simulink library "sm_interface_elements_lib"  (R2021b)
settings: Solver=VariableStepAuto  StartTime=0.0  StopTime=10.0  RelTol=1e-3
libraries: fl_lib x6, sm_lib x6
settings Model: Creator=The MathWorks, Inc.  LastModifiedBy=The MathWorks, Inc.
settings SolverCC: AlgebraicLoopSolver=TrustRegion
settings DebuggingCC: SFMachineParentedDataDiag=warning

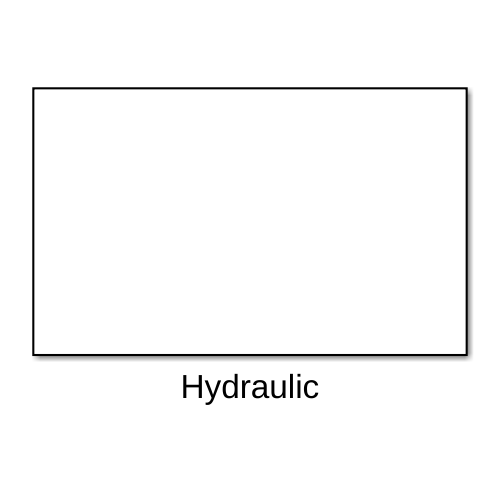
[thumbnail: Simulink's stored preview of the top-level diagram]
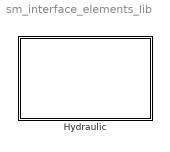
== system sm_interface_elements_lib ==
  Hydraulic : Subsystem
      mask init:
      | %

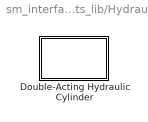
== system sm_interface_elements_lib/Hydraulic ==
  Double-Acting Hydraulic Cylinder : Subsystem  mask{barrelLength=0.5, barrelInnerRadius=0.08, barrelOuterRadius=0.1, barrelDensity=8050, barrelColor=[0.5 0.5 0.5], barrelOpacity=0.3, pistonThickness=0.05, pistonDensity=8050, pistonColor=[0.9 0.9 0.9], rodLength=0.5, rodRadius=0.04, rodDensity=8050, rodColor=[0.9 0.9 0.9], bottomCapThickness=0.05, bottomCapDensity=8050, bottomCapColor=[0.5 0.5 0.5], headCapThickness=0.05, headCapDensity=8050, headCapColor=[0.5 0.5 0.5], deadVolume_bottom=1e-6, deadVolume_head=1e-6, k_bottom=1e9, b_bottom=1500, k_head=1e9, b_head=1500, b=1e6, PositionTargetSpecify=on, PositionTargetPriority=Low (approximate), totalLength0=0.75, p0_bottom=4e6, p0_head=4e6}
      mask prompts: barrelLength "Length (m)"; barrelInnerRadius "Inner radius (m)"; barrelOuterRadius "Outer radius (m)"; barrelDensity "Density (kg/m^3)"; barrelColor "Color [R G B]"; barrelOpacity "Opacity"; pistonThickness "Thickness (m)"; pistonDensity "Density (kg/m^3)"; pistonColor "Color [R G B]"; rodLength "Length (m)"; rodRadius "Radius (m)"; rodDensity "Density (kg/m^3)"; rodColor "Color [R G B]"; bottomCapThickness "Thickness (m)"; bottomCapDensity "Density (kg/m^3)"; bottomCapColor "Color [R G B]"; headCapThickness "Thickness (m)"; headCapDensity "Density (kg/m^3)"; headCapColor "Color [R G B]"; deadVolume_bottom "Dead volume (m^3)"; deadVolume_head "Dead volume (m^3)"; k_bottom "Stiffness (N/m)"; b_bottom "Damping (N/(m/s))"; k_head "Stiffness (N/m)"; b_head "Damping (N/(m/s))"; b "Damping coefficient (N/m/s))"; PositionTargetSpecify "Specify end-to-end distance"; PositionTargetPriority "Priority"; totalLength0 "Bottom outer face to rod outer face distance (m)"; p0_bottom "Bottom chamber (Pa)"; p0_head "Head chamber (Pa)"
      mask help: This block represents a double-acting single-rod hydraulic cylinder. The 'head' end of the cylinder corresponds to the side through which the piston rod emerges. The block contains Simscape Multibody frame ports at the two ends: one attached to the outer face of the bottom end cap (FB) and the other attached to the outer face of the piston rod (FR). Hydraulic conserving ports are attached to the bottom chamber (HB) and the head chamber (HH).
      mask init:
      | blk = gcb;
      | 
      | % Piston face areas
      | pistonArea_bottom = pi*barrelInnerRadius^2;
      | pistonArea_head = pi*(barrelInnerRadius^2-rodRadius^2);
      | 
      | % Cylinder barrel cross section
      | barrelCrossSection = [...
      |     barrelInnerRadius,  barrelLength/2;...
      |     barrelInnerRadius, -barrelLength/2;...
      |     barrelOuterRadius, -barrelLength/2;...
      |     barrelOuterRadius,  barrelLength/2];
      | 
      | % Cylinder head cap cross section
      | headCapCrossSection = [...
      |     rodRadius,          headCapThickness/2;...
      |     rodRadius,         -headCapThickness/2;...
      |     barrelOuterRadius, -headCapThickness/2;...
      |     barrelOuterRadius,  headCapThickness/2];
      | 
      | % Set position target on Prismatic Joint
      | if PositionTargetSpecify
      |     set_param([blk,'/Mechanical System/Prismatic Joint'],'PositionTargetSpecify', 'on');
      |     length0_bottom = totalLength0 - rodLength - pistonThickness - bottomCapThickness;
      |     set_param([blk,'/Mechanical System/Prismatic Joint'],'PositionTargetValue', num2str(length0_bottom));
      |     switch PositionTargetPriority
      |         case 1 %'Low (approximate)'
      |             set_param([blk,'/Mechanical System/Prismatic Joint'],'PositionTargetPriority','Low');
      |         case 2 %'High (desired)'
      |             set_param([blk,'/Mechanical System/Prismatic Joint'],'PositionTargetPriority','High');
      |         otherwise
      |             disp('invalid target piority setting')
      |     end
      | else
      |     length0_bottom = 0;
      |     set_param([blk,'/Mechanical System/Prismatic Joint'],'PositionTargetSpecify', 'off');
      | end
      mask Callback PositionTargetSpecify:
      | simmechanics_demohelpers_dump_trailer_temp_mo = get_param(gcb,'MaskObject');
      | simmechanics_demohelpers_dump_trailer_temp_dc = simmechanics_demohelpers_dump_trailer_temp_mo.getDialogControl('PositionTargetParams');
      | if strcmp(get_param(gcb,'PositionTargetSpecify'),'on')
      |     simmechanics_demohelpers_dump_trailer_temp_dc.Visible = 'on';
      | else
      |     simmechanics_demohelpers_dump_trailer_temp_dc.Visible = 'off';
      | end
      | clear simmechanics_demohelpers_dump_trailer_temp_mo
      | clear simmechanics_demohelpers_dump_trailer_temp_dc
      mask TypeOptions PositionTargetPriority: Low (approximate) | High (desired)
      mask DialogControl Container4 Prompt: Bodies
      mask DialogControl Container30 Prompt: Cylinder Barrel
      mask DialogControl Container34 Prompt: Piston
      mask DialogControl Container35 Prompt: Rod
      mask DialogControl Container32 Prompt: Bottom Cap
      mask DialogControl Container33 Prompt: Head Cap
      mask DialogControl Container14 Prompt: Chambers
      mask DialogControl Container28 Prompt: Bottom
      mask DialogControl Container31 Prompt: Head
      mask DialogControl Container19 Prompt: Internal Mechanics
      mask DialogControl Container38 Prompt: Bottom Stop
      mask DialogControl Container41 Prompt: Head Stop
      mask DialogControl Container37 Prompt: Viscous Friction
      mask DialogControl Container25 Prompt: Initial Conditions
      mask DialogControl Container39 Prompt: Configuration
      mask DialogControl Container40 Prompt: Pressure
      mask Display: image(fullfile(matlabroot,'toolbox','physmod','sm','smdemos','interface_elements','images','sm_interface_elements_hydraulic_cylinder.svg'));

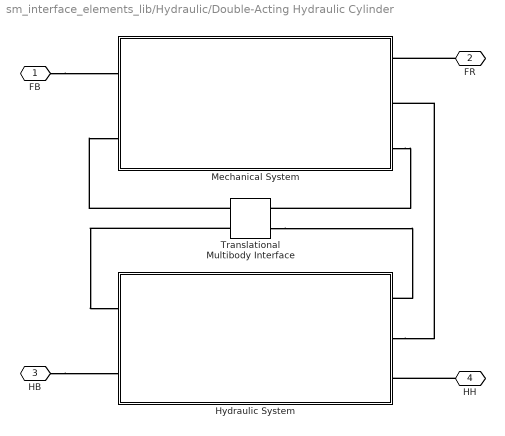
== system sm_interface_elements_lib/Hydraulic/Double-Acting Hydraulic Cylinder ==
  Hydraulic System : Subsystem
      mask Display: image(fullfile(matlabroot,'toolbox','physmod','sm','smdemos','dump_trailer','images','sm_dump_trailer_hydraulic_cylinder_hydraulic_system.svg'));
  Mechanical System : Subsystem
      mask Display: image(fullfile(matlabroot,'toolbox','physmod','sm','smdemos','dump_trailer','images','sm_dump_trailer_hydraulic_cylinder_mechanical_system.svg'));
  Translational Multibody Interface : fl_lib/Mechanical/Multibody Interfaces/Translational Multibody Interface
      settings: SourceProductBaseCode=SS
  FB : PMIOPort  Side=Left
  FR : PMIOPort  Port=2  Side=Right
  HB : PMIOPort  Port=3  Side=Left
  HH : PMIOPort  Port=4  Side=Right
  connections:
  FB/RConn1 -- Mechanical System/LConn1
  FR/RConn1 -- Mechanical System/RConn1
  HB/RConn1 -- Hydraulic System/LConn2
  HH/RConn1 -- Hydraulic System/RConn3
  Hydraulic System/RConn2 -- Mechanical System/RConn2
  Mechanical System/RConn3 -- Translational Multibody Interface/RConn1
  Translational Multibody Interface/LConn1 -- Mechanical System/LConn2
  Translational Multibody Interface/LConn2 -- Hydraulic System/LConn1
  Translational Multibody Interface/RConn2 -- Hydraulic System/RConn1

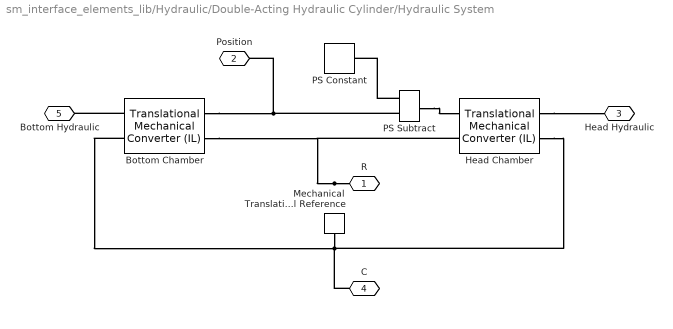
== system sm_interface_elements_lib/Hydraulic/Double-Acting Hydraulic Cylinder/Hydraulic System ==
  Bottom Chamber : fl_lib/Isothermal Liquid/Elements/Translational Mechanical Converter (IL)  mech_orientation=foundation.enum.MechOrientationTranslational.Positive  displacement_spec=foundation.enum.DisplacementSpec.InputSignal  x0=0 m  interface_area=pistonArea_bottom m^2  dead_volume=deadVolume_bottom m^3  pressure_spec=foundation.enum.pressure_spec.atmospheric  environment_pressure=0.101325 MPa  dynamic_compressibility=simscape.enum.onoff.on  p0=p0_bottom Pa
      settings: SourceProductBaseCode=SS  InternalSimscapePortConfiguration="{\"Bottom\":[],\"Left\":[{\"id\":\"A\",\"label\":\"A\",\"type\":\"foundation.isothermal_liquid.isothermal_liquid\"},{\"id\":\"C\",\"label\":\"C\",\"type\":\"foundation.mechanical.translational.translational\"}],\"Right\":[{\"id\":\"p_in\",\"label\":\"p\",\"type\":\"input\"},{\"id\":\"R\",\"label\":\"R\",\"type\":\"foundation.mechanical.translational.translational\"}],\"Top\":[]}"
  Head Chamber : fl_lib/Isothermal Liquid/Elements/Translational Mechanical Converter (IL)  mech_orientation=foundation.enum.MechOrientationTranslational.Negative  displacement_spec=foundation.enum.DisplacementSpec.InputSignal  x0=0 m  interface_area=pistonArea_head m^2  dead_volume=deadVolume_head m^3  pressure_spec=foundation.enum.pressure_spec.atmospheric  environment_pressure=0.101325 MPa  dynamic_compressibility=simscape.enum.onoff.on  p0=p0_head Pa
      settings: SourceProductBaseCode=SS  InternalSimscapePortConfiguration="{\"Bottom\":[],\"Left\":[{\"id\":\"A\",\"label\":\"A\",\"type\":\"foundation.isothermal_liquid.isothermal_liquid\"},{\"id\":\"C\",\"label\":\"C\",\"type\":\"foundation.mechanical.translational.translational\"}],\"Right\":[{\"id\":\"p_in\",\"label\":\"p\",\"type\":\"input\"},{\"id\":\"R\",\"label\":\"R\",\"type\":\"foundation.mechanical.translational.translational\"}],\"Top\":[]}"
  Mechanical Translational Reference : fl_lib/Mechanical/Translational Elements/Mechanical Translational Reference
  PS Constant : fl_lib/Physical Signals/Sources/PS Constant  constant=barrelLength-pistonThickness m
  PS Subtract : fl_lib/Physical Signals/Functions/PS Subtract
  R : PMIOPort  Side=Right
  Position : PMIOPort  Port=2  Side=Right
  Head Hydraulic : PMIOPort  Port=3  Side=Right
  C : PMIOPort  Port=4  Side=Left
  Bottom Hydraulic : PMIOPort  Port=5  Side=Left
  connections:
  Bottom Chamber/LConn1 -- Bottom Hydraulic/RConn1
  Head Chamber/LConn1 -- Head Hydraulic/RConn1
  PS Subtract/RConn1 -- Head Chamber/RConn1
  PS Subtract/LConn2 -- PS Constant/RConn1
  R/RConn1 -- Head Chamber/RConn2 -- Bottom Chamber/RConn2
  C/RConn1 -- Head Chamber/LConn2 -- Bottom Chamber/LConn2 -- Mechanical Translational Reference/LConn1
  Bottom Chamber/RConn1 -- PS Subtract/LConn1 -- Position/RConn1

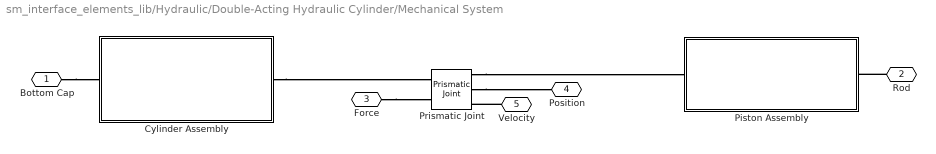
== system sm_interface_elements_lib/Hydraulic/Double-Acting Hydraulic Cylinder/Mechanical System ==
  Cylinder Assembly : Subsystem
      mask Display: image(fullfile(matlabroot,'toolbox','physmod','sm','smdemos','interface_elements','images','sm_interface_elements_hydraulic_cylinder_cylinder.png'));
  Piston Assembly : Subsystem
      mask Display: image(fullfile(matlabroot,'toolbox','physmod','sm','smdemos','interface_elements','images','sm_interface_elements_hydraulic_cylinder_piston.png'));
  Prismatic Joint : sm_lib/Joints/Prismatic Joint  JointMode=Normal  SenseConstraintForce=off  SenseConstraintForceX=off  SenseConstraintForceY=off  SenseConstraintForceZ=off  SenseConstraintTorque=off  SenseConstraintTorqueX=off  SenseConstraintTorqueY=off  SenseConstraintTorqueZ=off  SenseTotalForce=off  SenseTotalForceX=off  SenseTotalForceY=off  SenseTotalForceZ=off  SenseTotalTorque=off  SenseTotalTorqueX=off  SenseTotalTorqueY=off  SenseTotalTorqueZ=off  CompositeWrenchDir=FollowerOnBase  CompositeWrenchFrame=BaseFrame  EquilibriumPosition=0  EquilibriumPositionUnits=m  SpringStiffness=10  SpringStiffnessUnits=N/m  DampingCoefficient=b  DampingCoefficientUnits=N/(m/s)  TorqueActuationMode=InputTorque  MotionActuationMode=ComputedMotion  SensePosition=on  SenseVelocity=on  SenseAcceleration=off  SenseTorqueForce=off  SenseLowerLimitTorqueForce=off  SenseUpperLimitTorqueForce=off  LowerLimitSpecify=on  LowerLimitBound=0  LowerLimitBoundUnits=m  LowerLimitStiffness=k_bottom  LowerLimitStiffnessUnits=N/m  LowerLimitDamping=b_bottom  LowerLimitDampingUnits=N/(m/s)  LowerLimitTransitionRegionWidth=1e-4  LowerLimitTransitionRegionWidthUnits=m  UpperLimitSpecify=on  UpperLimitBound=barrelLength-pistonThickness  UpperLimitBoundUnits=m  UpperLimitStiffness=k_head  UpperLimitStiffnessUnits=N/m  UpperLimitDamping=b_head  UpperLimitDampingUnits=N/(m/s)  UpperLimitTransitionRegionWidth=1e-4  UpperLimitTransitionRegionWidthUnits=m  PositionTargetSpecify=on  PositionTargetPriority=Low  PositionTargetValue=0.15  PositionTargetValueUnits=m  VelocityTargetSpecify=off  VelocityTargetPriority=High  VelocityTargetValue=0  VelocityTargetValueUnits=m/s
  Bottom Cap : PMIOPort  Side=Left
  Rod : PMIOPort  Port=2  Side=Right
  Force : PMIOPort  Port=3  Side=Left
  Position : PMIOPort  Port=4  Side=Right
  Velocity : PMIOPort  Port=5  Side=Right
  connections:
  Bottom Cap/RConn1 -- Cylinder Assembly/LConn1
  Rod/RConn1 -- Piston Assembly/RConn1
  Cylinder Assembly/RConn1 -- Prismatic Joint/LConn1
  Prismatic Joint/RConn1 -- Piston Assembly/LConn1
  Prismatic Joint/RConn2 -- Position/RConn1
  Force/RConn1 -- Prismatic Joint/LConn2
  Velocity/RConn1 -- Prismatic Joint/RConn3

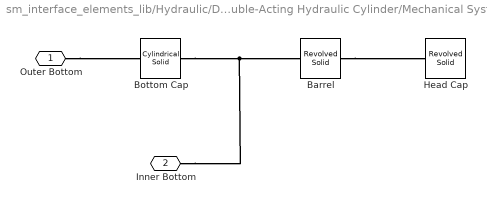
== system sm_interface_elements_lib/Hydraulic/Double-Acting Hydraulic Cylinder/Mechanical System/Cylinder Assembly ==
  Barrel : sm_lib/Body Elements/Revolved Solid  GraphicAmbientColor=[0.15 0.15 0.15 1.0]  BasedOnType=Density  CenterOfMass=[0 0 0]  CenterOfMassUnits=m  GraphicDiffuseColor=barrelColor  ExportConvexHullGeometry=off  Density=barrelDensity  DensityUnits=kg/m^3  DoExposeReferenceFrame=off  GraphicEmissiveColor=[0.0 0.0 0.0 1.0]  ExportEntireGeometry=off  SerializedFrames=<Frames><Frame><Id>Frame1</Id><Value><Name>left</Name><Origin><Source>GeometricFeature</Source><FeatureName>side curve 3</FeatureName></Origin><PrimaryAxis><DefinedDirection>+Z</DefinedDirection><Source>ReferenceFrame</Source><SourceDirection>+Z</SourceDirection><FeatureName></FeatureName></PrimaryAxis><SecondaryAxis><DefinedDirection>+X</DefinedDirection><Source>ReferenceFrame</Source><SourceDirection>+X</SourceDirection><FeatureName></FeatureName></SecondaryAxis></Value></Frame><Frame><Id>Frame2</Id><Value><Name>right</Name><Origin><Source>GeometricFeature</Source><FeatureName>side curve 4</FeatureName></Origin><PrimaryAxis><DefinedDirection>+Z</DefinedDirection><Source>ReferenceFrame</Source><SourceDirection>-Z</SourceDirection><FeatureName></FeatureName></PrimaryAxis><SecondaryAxis><DefinedDirection>+Y</DefinedDirection><Source>ReferenceFrame</Source><SourceDirection>+Y</SourceDirection><FeatureName></FeatureName></SecondaryAxis></Value></Frame></Frames>  MarkerShape=Sphere  MarkerSize=10  GraphicType=FromGeometry  InertiaType=CalculateFromGeometry  Mass=1  MassUnits=kg  MomentsOfInertia=[1 1 1]  MomentsOfInertiaUnits=kg*m^2  GraphicOpacity=barrelOpacity  ProductsOfInertia=[0 0 0]  ProductsOfInertiaUnits=kg*m^2  RevolutionCrossSection=barrelCrossSection  RevolutionCrossSectionUnits=m  RevolutionAngle=180  RevolutionAngleUnits=deg  RevolutionExtent=Full  GraphicShininess=75  GraphicSpecularColor=[0.5 0.5 0.5 1.0]  GraphicVisPropType=SimpleVisualProperties
  Bottom Cap : sm_lib/Body Elements/Cylindrical Solid  GraphicAmbientColor=[0.15 0.15 0.15 1.0]  BasedOnType=Density  CenterOfMass=[0 0 0]  CenterOfMassUnits=m  GraphicDiffuseColor=bottomCapColor  CylinderLength=bottomCapThickness  CylinderLengthUnits=m  CylinderRadius=barrelOuterRadius  CylinderRadiusUnits=m  Density=bottomCapDensity  DensityUnits=kg/m^3  DoExposeReferenceFrame=off  GraphicEmissiveColor=[0.0 0.0 0.0 1.0]  ExportEntireGeometry=off  SerializedFrames=<Frames><Frame><Id>Frame1</Id><Value><Name>left</Name><Origin><Source>GeometricFeature</Source><FeatureName>bottom surface</FeatureName></Origin><PrimaryAxis><DefinedDirection>+Z</DefinedDirection><Source>ReferenceFrame</Source><SourceDirection>-Z</SourceDirection><FeatureName></FeatureName></PrimaryAxis><SecondaryAxis><DefinedDirection>+Y</DefinedDirection><Source>ReferenceFrame</Source><SourceDirection>+Y</SourceDirection><FeatureName></FeatureName></SecondaryAxis></Value></Frame><Frame><Id>Frame2</Id><Value><Name>right</Name><Origin><Source>GeometricFeature</Source><FeatureName>top surface</FeatureName></Origin><PrimaryAxis><DefinedDirection>+Z</DefinedDirection><Source>ReferenceFrame</Source><SourceDirection>+Z</SourceDirection><FeatureName></FeatureName></PrimaryAxis><SecondaryAxis><DefinedDirection>+X</DefinedDirection><Source>ReferenceFrame</Source><SourceDirection>+X</SourceDirection><FeatureName></FeatureName></SecondaryAxis></Value></Frame></Frames>  MarkerShape=Sphere  MarkerSize=10  GraphicType=FromGeometry  InertiaType=CalculateFromGeometry  Mass=1  MassUnits=kg  MomentsOfInertia=[1 1 1]  MomentsOfInertiaUnits=kg*m^2  GraphicOpacity=1  ProductsOfInertia=[0 0 0]  ProductsOfInertiaUnits=kg*m^2  GraphicShininess=75  GraphicSpecularColor=[0.5 0.5 0.5 1.0]  GraphicVisPropType=SimpleVisualProperties
  Head Cap : sm_lib/Body Elements/Revolved Solid  GraphicAmbientColor=[0.15 0.15 0.15 1.0]  BasedOnType=Density  CenterOfMass=[0 0 0]  CenterOfMassUnits=m  GraphicDiffuseColor=headCapColor  ExportConvexHullGeometry=off  Density=headCapDensity  DensityUnits=kg/m^3  DoExposeReferenceFrame=off  GraphicEmissiveColor=[0.0 0.0 0.0 1.0]  ExportEntireGeometry=off  SerializedFrames=<Frames><Frame><Id>Frame1</Id><Value><Name>left</Name><Origin><Source>GeometricFeature</Source><FeatureName>side surface 2</FeatureName></Origin><PrimaryAxis><DefinedDirection>+Z</DefinedDirection><Source>ReferenceFrame</Source><SourceDirection>-Z</SourceDirection><FeatureName></FeatureName></PrimaryAxis><SecondaryAxis><DefinedDirection>+Y</DefinedDirection><Source>ReferenceFrame</Source><SourceDirection>+Y</SourceDirection><FeatureName></FeatureName></SecondaryAxis></Value></Frame></Frames>  MarkerShape=Sphere  MarkerSize=10  GraphicType=FromGeometry  InertiaType=CalculateFromGeometry  Mass=1  MassUnits=kg  MomentsOfInertia=[1 1 1]  MomentsOfInertiaUnits=kg*m^2  GraphicOpacity=1.0  ProductsOfInertia=[0 0 0]  ProductsOfInertiaUnits=kg*m^2  RevolutionCrossSection=headCapCrossSection  RevolutionCrossSectionUnits=m  RevolutionAngle=180  RevolutionAngleUnits=deg  RevolutionExtent=Full  GraphicShininess=75  GraphicSpecularColor=[0.5 0.5 0.5 1.0]  GraphicVisPropType=SimpleVisualProperties
  Outer Bottom : PMIOPort  Side=Left
  Inner Bottom : PMIOPort  Port=2  Side=Right
  connections:
  Inner Bottom/RConn1 -- Bottom Cap/RConn1 -- Barrel/LConn1
  Barrel/RConn1 -- Head Cap/LConn1
  Outer Bottom/RConn1 -- Bottom Cap/LConn1

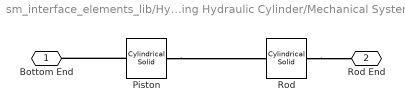
== system sm_interface_elements_lib/Hydraulic/Double-Acting Hydraulic Cylinder/Mechanical System/Piston Assembly ==
  Piston : sm_lib/Body Elements/Cylindrical Solid  GraphicAmbientColor=[0.15 0.15 0.15 1.0]  BasedOnType=Density  CenterOfMass=[0 0 0]  CenterOfMassUnits=m  GraphicDiffuseColor=pistonColor  CylinderLength=pistonThickness  CylinderLengthUnits=m  CylinderRadius=barrelInnerRadius  CylinderRadiusUnits=m  Density=pistonDensity  DensityUnits=kg/m^3  DoExposeReferenceFrame=off  GraphicEmissiveColor=[0.0 0.0 0.0 1.0]  ExportEntireGeometry=off  SerializedFrames=<Frames><Frame><Id>Frame1</Id><Value><Name>left</Name><Origin><Source>GeometricFeature</Source><FeatureName>bottom surface</FeatureName></Origin><PrimaryAxis><DefinedDirection>+Z</DefinedDirection><Source>ReferenceFrame</Source><SourceDirection>+Z</SourceDirection><FeatureName></FeatureName></PrimaryAxis><SecondaryAxis><DefinedDirection>+X</DefinedDirection><Source>ReferenceFrame</Source><SourceDirection>+X</SourceDirection><FeatureName></FeatureName></SecondaryAxis></Value></Frame><Frame><Id>Frame2</Id><Value><Name>right</Name><Origin><Source>GeometricFeature</Source><FeatureName>top surface</FeatureName></Origin><PrimaryAxis><DefinedDirection>+Z</DefinedDirection><Source>ReferenceFrame</Source><SourceDirection>+Z</SourceDirection><FeatureName></FeatureName></PrimaryAxis><SecondaryAxis><DefinedDirection>+X</DefinedDirection><Source>ReferenceFrame</Source><SourceDirection>+X</SourceDirection><FeatureName></FeatureName></SecondaryAxis></Value></Frame></Frames>  MarkerShape=Sphere  MarkerSize=10  GraphicType=FromGeometry  InertiaType=CalculateFromGeometry  Mass=1  MassUnits=kg  MomentsOfInertia=[1 1 1]  MomentsOfInertiaUnits=kg*m^2  GraphicOpacity=1.0  ProductsOfInertia=[0 0 0]  ProductsOfInertiaUnits=kg*m^2  GraphicShininess=75  GraphicSpecularColor=[0.5 0.5 0.5 1.0]  GraphicVisPropType=SimpleVisualProperties
  Rod : sm_lib/Body Elements/Cylindrical Solid  GraphicAmbientColor=[0.15 0.15 0.15 1.0]  BasedOnType=Density  CenterOfMass=[0 0 0]  CenterOfMassUnits=m  GraphicDiffuseColor=rodColor  CylinderLength=rodLength  CylinderLengthUnits=m  CylinderRadius=rodRadius  CylinderRadiusUnits=m  Density=rodDensity  DensityUnits=kg/m^3  DoExposeReferenceFrame=off  GraphicEmissiveColor=[0.0 0.0 0.0 1.0]  ExportEntireGeometry=off  SerializedFrames=<Frames><Frame><Id>Frame1</Id><Value><Name>left</Name><Origin><Source>GeometricFeature</Source><FeatureName>bottom surface</FeatureName></Origin><PrimaryAxis><DefinedDirection>+Z</DefinedDirection><Source>ReferenceFrame</Source><SourceDirection>+Z</SourceDirection><FeatureName></FeatureName></PrimaryAxis><SecondaryAxis><DefinedDirection>+X</DefinedDirection><Source>ReferenceFrame</Source><SourceDirection>+X</SourceDirection><FeatureName></FeatureName></SecondaryAxis></Value></Frame><Frame><Id>Frame2</Id><Value><Name>right</Name><Origin><Source>GeometricFeature</Source><FeatureName>top surface</FeatureName></Origin><PrimaryAxis><DefinedDirection>+Z</DefinedDirection><Source>ReferenceFrame</Source><SourceDirection>+Z</SourceDirection><FeatureName></FeatureName></PrimaryAxis><SecondaryAxis><DefinedDirection>+X</DefinedDirection><Source>ReferenceFrame</Source><SourceDirection>+X</SourceDirection><FeatureName></FeatureName></SecondaryAxis></Value></Frame></Frames>  MarkerShape=Sphere  MarkerSize=10  GraphicType=FromGeometry  InertiaType=CalculateFromGeometry  Mass=1  MassUnits=kg  MomentsOfInertia=[1 1 1]  MomentsOfInertiaUnits=kg*m^2  GraphicOpacity=1.0  ProductsOfInertia=[0 0 0]  ProductsOfInertiaUnits=kg*m^2  GraphicShininess=75  GraphicSpecularColor=[0.5 0.5 0.5 1.0]  GraphicVisPropType=AdvancedVisualProperties
  Bottom End : PMIOPort  Side=Left
  Rod End : PMIOPort  Port=2  Side=Right
  connections:
  Piston/LConn1 -- Bottom End/RConn1
  Piston/RConn1 -- Rod/LConn1
  Rod/RConn1 -- Rod End/RConn1
